simulink model "FA_18_Model_2016"  (R2016b)
settings: Solver=ode45  StartTime=0.0  StopTime=600  FixedStep=0.1  MaxStep=0.1  RelTol=1e-3
PreLoadFcn:
  | load('FA_18_Parameters.mat')
  | format long
undefined symbols (not defined in the file or in its folder): Earth, WGS84
libraries: aerolibfltsims x2, aerolibtransform2 x1, aerolibconvert2 x1
settings Model: Creator=User  LastModifiedBy=User

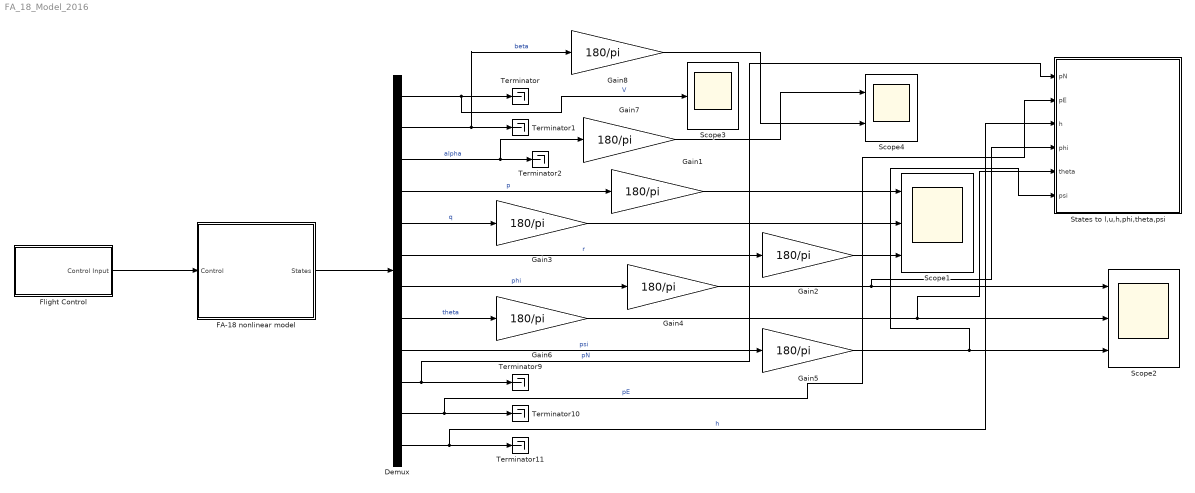
== system FA_18_Model_2016 ==
  Demux : Demux  Outputs=12
  FA-18 nonlinear model : Subsystem
  Flight Control : Subsystem
  Gain{1..3,5..8} (7 alike) : Gain  Gain=180/pi
  Gain4 : Gain  Gain=180/pi  ParamDataTypeStr=double  OutDataTypeStr=double
  Scope1 : Scope  NumInputPorts=3
  Scope2 : Scope  NumInputPorts=3
  Scope3 : Scope
  Scope4 : Scope  NumInputPorts=2
  States to l,u,h,phi,theta,psi : Subsystem
  Terminator{,1..2,9..11} (6 alike) : Terminator
  wires:
  Demux/3 -> Gain7/1, Terminator2/1  "alpha"
  Demux/2 -> Terminator1/1, Gain8/1  "beta"
  Demux/1 -> Scope3/1, Terminator/1  "V"
  Demux/7 -> Gain4/1  "phi"
  Demux/4 -> Gain1/1  "p"
  Demux/10 -> States to l,u,h,phi,theta,psi/1(pN), Terminator9/1  "pN"
  FA-18 nonlinear model/1(States) -> Demux/1
  Demux/11 -> States to l,u,h,phi,theta,psi/2(pE), Terminator10/1  "pE"
  Demux/6 -> Gain2/1  "r"
  Demux/12 -> States to l,u,h,phi,theta,psi/3(h), Terminator11/1  "h"
  Demux/5 -> Gain3/1  "q"
  Gain1/1 -> Scope1/1
  Gain2/1 -> Scope1/3
  Gain3/1 -> Scope1/2
  Gain4/1 -> States to l,u,h,phi,theta,psi/4(phi), Scope2/1
  Gain5/1 -> States to l,u,h,phi,theta,psi/6(psi), Scope2/3
  Gain6/1 -> States to l,u,h,phi,theta,psi/5(theta), Scope2/2
  Demux/8 -> Gain6/1  "theta"
  Demux/9 -> Gain5/1  "psi"
  Flight Control/1(Control Input) -> FA-18 nonlinear model/1(Control)
  Gain7/1 -> Scope4/1
  Gain8/1 -> Scope4/2

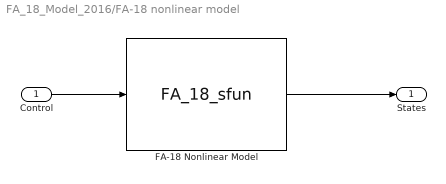
== system FA_18_Model_2016/FA-18 nonlinear model ==
  Control : Inport
  FA-18 Nonlinear Model : S-Function  FunctionName=FA_18_sfun  SFunctionDeploymentMode=off  EnableBusSupport=off
  States : Outport
  wires:
  FA-18 Nonlinear Model/1 -> States/1
  Control/1 -> FA-18 Nonlinear Model/1

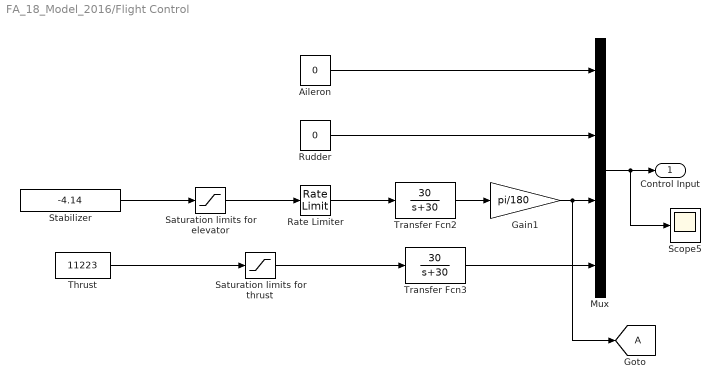
== system FA_18_Model_2016/Flight Control ==
  Aileron : Constant  Value=0
  Gain1 : Gain  Gain=pi/180
  Mux : Mux
  Rate Limiter : RateLimiter  RisingSlewLimit=40  FallingSlewLimit=-40  SampleTimeMode=inherited
  Rudder : Constant  Value=0
  Saturation limits for elevator : Saturate  UpperLimit=10.5  LowerLimit=-24
  Saturation limits for thrust : Saturate  UpperLimit=20000  LowerLimit=0
  Scope5 : Scope
  Stabilizer : Constant  Value=-4.14
  Thrust : Constant  Value=11223
  Transfer Fcn2 : TransferFcn  Numerator=[30]  Denominator=[1 30]
  Transfer Fcn3 : TransferFcn  Numerator=[30]  Denominator=[1 30]
  Control Input : Outport
  tag scope: A=global
  wires:
  Mux/1 -> Scope5/1, Control Input/1
  Aileron/1 -> Mux/1
  Thrust/1 -> Saturation limits for thrust/1
  Transfer Fcn3/1 -> Mux/4
  Rudder/1 -> Mux/2
  Saturation limits for thrust/1 -> Transfer Fcn3/1
  Saturation limits for elevator/1 -> Rate Limiter/1
  Rate Limiter/1 -> Transfer Fcn2/1
  Stabilizer/1 -> Saturation limits for elevator/1
  Gain1/1 -> [A], Mux/3
  Transfer Fcn2/1 -> Gain1/1

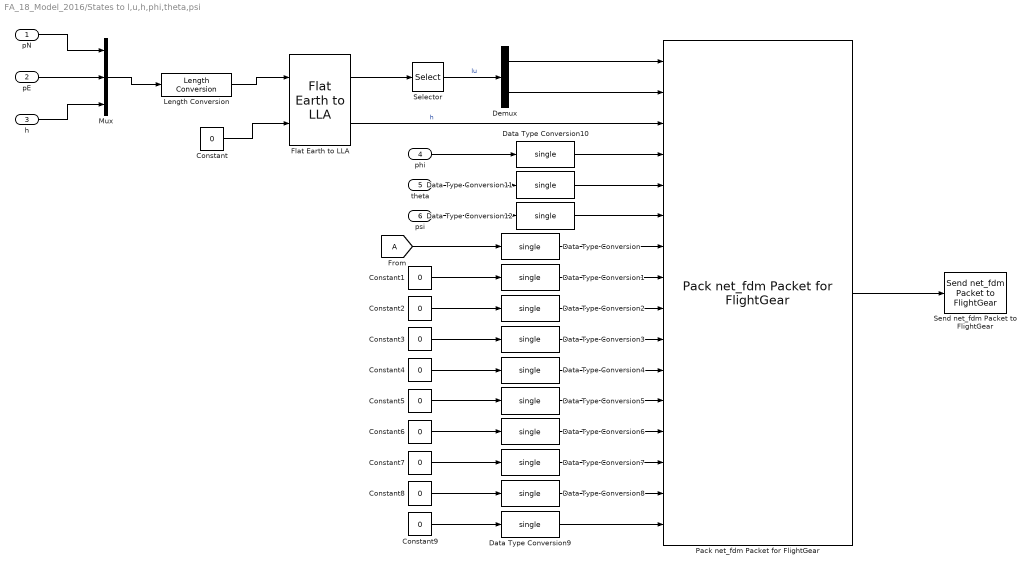
== system FA_18_Model_2016/States to l,u,h,phi,theta,psi ==
  pN : Inport
  pE : Inport  Port=2
  h : Inport  Port=3
  phi : Inport  Port=4
  theta : Inport  Port=5
  psi : Inport  Port=6
  Constant{,2..9} (9 alike) : Constant  Value=0
  Constant1 : Constant  Value=0  OutDataTypeStr=single
  Data Type Conversion{,1..12} (13 alike) : DataTypeConversion  OutDataTypeStr=single
  Demux : Demux  Outputs=2
  Flat Earth to LLA : aerolibtransform2/Flat Earth to LLA  units=Metric (MKS)  ptype=Earth (WGS84)  F=1/298.257223563  R=6378137  LL0=[50.1018 14.2632]  psi=0
  Length Conversion : aerolibconvert2/Length Conversion  IU=ft  OU=m
  Mux : Mux  Inputs=3
  Pack net_fdm Packet for FlightGear : aerolibfltsims/Pack net_fdm Packet for FlightGear  FlightGearVersion=v2017.3  ShowPositionAttitudeInputs=on  ShowVelocityAccelerationInputs=off  ShowControlSurfacePositionInputs=on  ShowEngineFuelInputs=off  ShowLandingGearInputs=off  ShowEnvironmentInputs=off  SampleTime=1/30
  Selector : Selector  IndexMode=Zero-based  InputPortWidth=2  IndexOptions=Index vector (dialog)  Indices=[1 0]  OutputSizes=1
  Send net_fdm Packet to FlightGear : aerolibfltsims/Send net_fdm Packet to FlightGear  DestinationIpAddress=127.0.0.1  DestinationPort=5502  LocalIpPort=-1  varLen=off  SampleTime=1/30
  wires:
  Constant/1 -> Flat Earth to LLA/2
  Length Conversion/1 -> Flat Earth to LLA/1
  Flat Earth to LLA/1 -> Selector/1
  Selector/1 -> Demux/1  "lu"
  Flat Earth to LLA/2 -> Pack net_fdm Packet for FlightGear/3  "h"
  pN/1 -> Mux/1
  pE/1 -> Mux/2
  h/1 -> Mux/3
  Mux/1 -> Length Conversion/1
  theta/1 -> Data Type Conversion11/1
  phi/1 -> Data Type Conversion10/1
  Pack net_fdm Packet for FlightGear/1 -> Send net_fdm Packet to FlightGear/1
  psi/1 -> Data Type Conversion12/1
  Constant1/1 -> Data Type Conversion1/1
  Constant2/1 -> Data Type Conversion2/1
  Constant3/1 -> Data Type Conversion3/1
  Constant4/1 -> Data Type Conversion4/1
  Constant5/1 -> Data Type Conversion5/1
  Constant6/1 -> Data Type Conversion6/1
  Constant7/1 -> Data Type Conversion7/1
  Constant8/1 -> Data Type Conversion8/1
  Constant9/1 -> Data Type Conversion9/1
  [A] -> Data Type Conversion/1
  Data Type Conversion/1 -> Pack net_fdm Packet for FlightGear/7
  Data Type Conversion1/1 -> Pack net_fdm Packet for FlightGear/8
  Data Type Conversion2/1 -> Pack net_fdm Packet for FlightGear/9
  Data Type Conversion3/1 -> Pack net_fdm Packet for FlightGear/10
  Data Type Conversion4/1 -> Pack net_fdm Packet for FlightGear/11
  Data Type Conversion5/1 -> Pack net_fdm Packet for FlightGear/12
  Data Type Conversion6/1 -> Pack net_fdm Packet for FlightGear/13
  Data Type Conversion7/1 -> Pack net_fdm Packet for FlightGear/14
  Data Type Conversion8/1 -> Pack net_fdm Packet for FlightGear/15
  Data Type Conversion9/1 -> Pack net_fdm Packet for FlightGear/16
  Data Type Conversion10/1 -> Pack net_fdm Packet for FlightGear/4
  Data Type Conversion11/1 -> Pack net_fdm Packet for FlightGear/5
  Data Type Conversion12/1 -> Pack net_fdm Packet for FlightGear/6
  Demux/2 -> Pack net_fdm Packet for FlightGear/2
  Demux/1 -> Pack net_fdm Packet for FlightGear/1
